simulink model "rl_sin"  (R2017b)
settings: Solver=ode23tb  StartTime=0.0  StopTime=0.2  RelTol=1e-3  EnableMultiTasking=on
values from neighbouring files (symbols this model uses):
  L = 0.05    [task1.m]
  R = 2    [task1.m]
  Ts = 0.002    [task1.m]
  Udc = 600    [task1.m]
  Uftopp = sqrt(2)*230    [task1.m]
settings Model: Creator=ielolof  LastModifiedBy=Morten
settings DataIOCC: SaveFormat=Array  SignalLoggingSaveFormat=ModelDataLogs  TimeSaveName=tpwm
settings OptimizationCC: ExpressionDepthLimit=2147483647  InitFltsAndDblsToZero=on  LifeSpan=inf
settings DebuggingCC: UnderspecifiedInitializationDetection=Classic  MergeDetectMultiDrivingBlocksExec=none  SolverPrmCheckMsg=warning  FcnCallInpInsideContextMsg=warning  StateNameClashWarn=warning  StrictBusMsg=Warning  SFUnexpectedBacktrackingDiag=warning  SFNoUnconditionalDefaultTransitionDiag=warning  SFExecutionAtInitializationDiag=none
settings HardwareCC: ProdBitPerPointer=32  ProdBitPerSizeT=32  ProdBitPerPtrDiffT=32  ProdLargestAtomicFloat=None  ProdIntDivRoundTo=Undefined  ProdEndianess=Unspecified  ProdWordSize=32  ProdHWDeviceType=32-bit Generic
settings ModelReferenceCC: PropagateSignalLabelsOutOfModel=off
settings CodeAppCC: StateflowObjectComments=on
settings GRTTargetCC: TargetLangStandard=C89/C90 (ANSI)  CombineOutputUpdateFcns=off  GRTInterface=on
settings ConfigComp: CovMetricSettings=dw  CovHtmlReporting=on  CovSaveCumulativeToWorkspaceVar=on  CovSaveSingleToWorkspaceVar=on  CovExternalEMLEnable=off

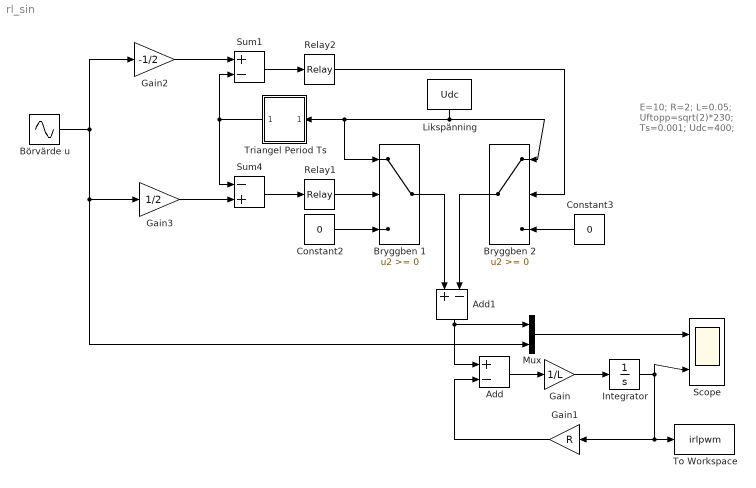
== system rl_sin ==
  note: E=10;
      | R=2;
      | L=0.05;
      |
      | Uftopp=sqrt(2)*230;
      | Ts=0.001;
      | Udc=400;
  Add : Sum  Inputs=+-
  Add1 : Sum  Inputs=+-
  Bryggben 1 : Switch  SaturateOnIntegerOverflow=on  InputSameDT=on
  Bryggben 2 : Switch  SaturateOnIntegerOverflow=on  InputSameDT=on
  Börvärde u : Sin  Amplitude=Uftopp  Frequency=100*pi  SampleTime=0
  Constant2 : Constant  Value=0
  Constant3 : Constant  Value=0
  Gain : Gain  Gain=1/L
  Gain1 : Gain  Gain=R
  Gain2 : Gain  Gain=-1/2
  Gain3 : Gain  Gain=1/2
  Integrator : Integrator
  Likspänning : Constant  Value=Udc
  Mux : Mux  Inputs=2
  Relay1 : Relay  OffOutputValue=-1
  Relay2 : Relay  OffOutputValue=-1
  Scope : Scope  NumInputPorts=2
  Sum1 : Sum  Inputs=+-  SaturateOnIntegerOverflow=on  InputSameDT=on  OutDataTypeStr=Inherit: Same as first input
  Sum4 : Sum  Inputs=-+  SaturateOnIntegerOverflow=on  InputSameDT=on  OutDataTypeStr=Inherit: Same as first input
  To Workspace : ToWorkspace  VariableName=irlpwm  SampleTime=-1
  Triangel Period Ts : Subsystem
  wires:
  Add/1 -> Gain/1
  Gain/1 -> Integrator/1
  Integrator/1 -> Gain1/1, To Workspace/1, Scope/2
  Gain1/1 -> Add/2
  Likspänning/1 -> Bryggben 1/1, Triangel Period Ts/1(Udc), Bryggben 2/1
  Constant2/1 -> Bryggben 1/3
  Börvärde u/1 -> Gain3/1, Mux/2, Gain2/1
  Sum4/1 -> Relay1/1
  Relay1/1 -> Bryggben 1/2
  Triangel Period Ts/1(um) -> Sum4/1, Sum1/2
  Bryggben 1/1 -> Add1/1
  Bryggben 2/1 -> Add1/2
  Add1/1 -> Add/1, Mux/1
  Constant3/1 -> Bryggben 2/3
  Relay2/1 -> Bryggben 2/2
  Sum1/1 -> Relay2/1
  Gain3/1 -> Sum4/2
  Gain2/1 -> Sum1/1
  Mux/1 -> Scope/1

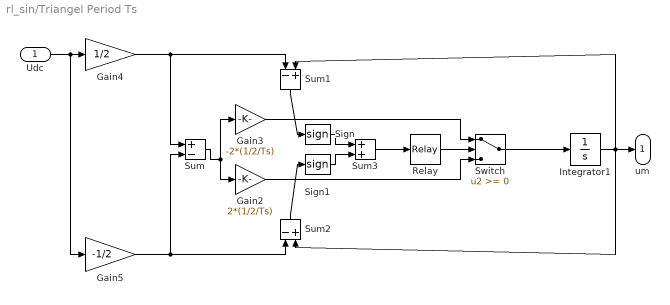
== system rl_sin/Triangel Period Ts ==
  Udc : Inport
  Gain2 : Gain  Gain=2*(1/2/Ts)  SaturateOnIntegerOverflow=on  OutDataTypeStr=Inherit: Same as input  ParamDataTypeStr=Inherit: Same as input
  Gain3 : Gain  Gain=-2*(1/2/Ts)  SaturateOnIntegerOverflow=on  OutDataTypeStr=Inherit: Same as input  ParamDataTypeStr=Inherit: Same as input
  Gain4 : Gain  Gain=1/2  SaturateOnIntegerOverflow=on  OutDataTypeStr=Inherit: Same as input  ParamDataTypeStr=Inherit: Same as input
  Gain5 : Gain  Gain=-1/2  SaturateOnIntegerOverflow=on  OutDataTypeStr=Inherit: Same as input  ParamDataTypeStr=Inherit: Same as input
  Integrator1 : Integrator
  Relay : Relay  OnSwitchValue=1  OffSwitchValue=-1  OffOutputValue=-1
  Sign : Signum
  Sign1 : Signum
  Sum : Sum  Inputs=+-  SaturateOnIntegerOverflow=on  InputSameDT=on  OutDataTypeStr=Inherit: Same as first input
  Sum1 : Sum  Inputs=-+  SaturateOnIntegerOverflow=on  InputSameDT=on  OutDataTypeStr=Inherit: Same as first input
  Sum2 : Sum  Inputs=-+  SaturateOnIntegerOverflow=on  InputSameDT=on  OutDataTypeStr=Inherit: Same as first input
  Sum3 : Sum  SaturateOnIntegerOverflow=on  InputSameDT=on  OutDataTypeStr=Inherit: Same as first input
  Switch : Switch  SaturateOnIntegerOverflow=on  InputSameDT=on
  um : Outport
  wires:
  Switch/1 -> Integrator1/1
  Gain3/1 -> Switch/1
  Gain2/1 -> Switch/3
  Integrator1/1 -> Sum1/2, Sum2/2, um/1
  Sum1/1 -> Sign/1
  Sum2/1 -> Sign1/1
  Sign/1 -> Sum3/1
  Sign1/1 -> Sum3/2
  Sum3/1 -> Relay/1
  Relay/1 -> Switch/2
  Sum/1 -> Gain3/1, Gain2/1
  Udc/1 -> Gain5/1, Gain4/1
  Gain5/1 -> Sum/2, Sum2/1
  Gain4/1 -> Sum/1, Sum1/1
